simulink model "ModuleCooling"  (R2024b)
settings: Solver=VariableStepAuto  StartTime=0.0  StopTime=800  RelTol=1e-3
PostLoadFcn:
  | pouchPackExample_param;
  | load Artemis150mphCurrent_TS.mat;
undefined symbols (not defined in the file or in its folder): battery_builder_rtmsupport, gcbh
libraries: fl_lib x7, nesl_utility x6, batt_lib x2, pouchPackExample_lib x1, SimscapeFluids_lib x1
settings Model: Creator=xiangchz  LastModifiedBy=xiangchz
settings OptimizationCC: ReuseModelBlockBuffer=off
settings RTWCC: GPUComputeCapability=3.5
settings SimscapeCC: SimscapeLogType=all

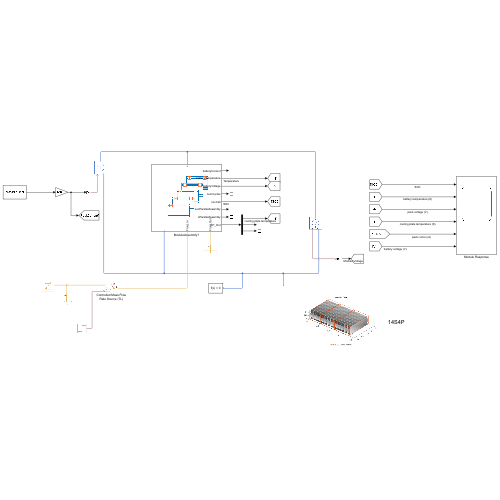
[thumbnail: Simulink's stored preview of the top-level diagram]
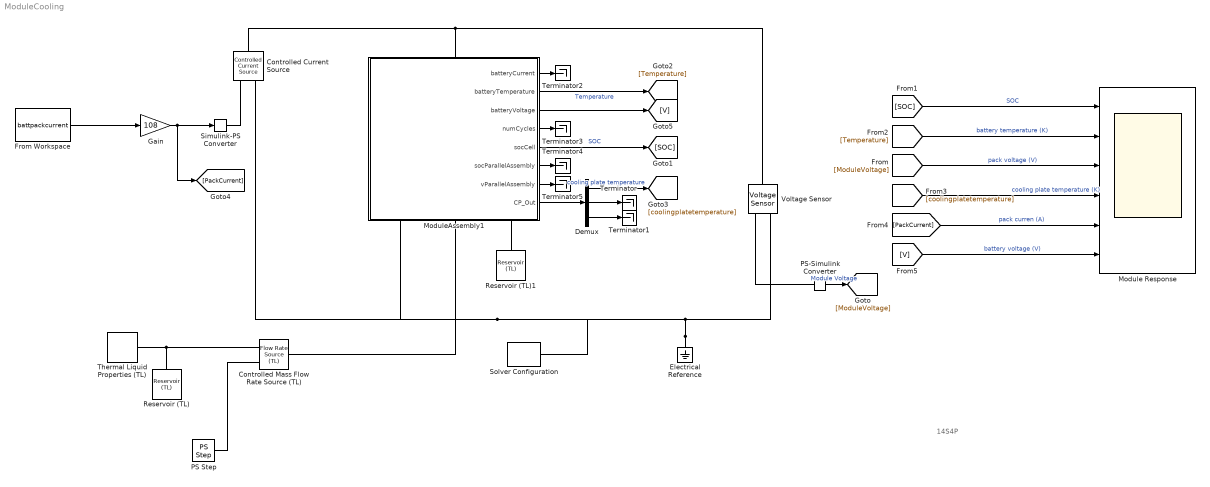
== system ModuleCooling ==
  note: 14S4P
  Controlled Current Source : fl_lib/Electrical/Electrical Sources/Controlled Current Source
  Controlled Mass Flow Rate Source (TL) : fl_lib/Thermal Liquid/Sources/Flow Rate Source (TL)  source_type=foundation.enum.constant_controlled.controlled  flow_type=foundation.enum.mass_volumetric_flow.mass  mass_flow=0 kg/s  volumetric_flow=0 m^3/s  power_spec=foundation.enum.power_spec.isentropic  area=0.01 m^2
  Demux : Demux  Outputs=[10 1 1]
  Electrical Reference : fl_lib/Electrical/Electrical Elements/Electrical Reference
  From Workspace : FromWorkspace  VariableName=battpackcurrent  OutputAfterFinalValue=Setting to zero
  Gain : Gain  Gain=108
  Module Response : Scope  NumInputPorts=6
  ModuleAssembly1 : Subsystem  LoadFcn=battery_builder_rtmsupport('loadfcn',gcbh);
      settings: CopyFcn=battery_builder_rtmsupport('copyfcn',gcbh);  PreCopyFcn=battery_builder_rtmsupport('precopyfcn',gcbh);  PreDeleteFcn=battery_builder_rtmsupport('predeletefcn',gcbh);  PortSchema="{\"entries\":[{\"content\":{\"sides\":[{\"content\":{\"connectorIds\":[\"LConn1\"]},\"type\":\"ConnectorPlacement.EquallySpacedRectSide\",\"uuid\":\"a5a584e8-f613-435c-beac-db0de62ed6e0\"},{\"content\":{\"connectorIds\":[\"RConn1\",\"RConn2\",\"RConn3\"],\"side\":\"RIGHT\"},\"type\":\"ConnectorPlacement.EquallySpacedRectSide\",\"uuid\":\"d51acd9b-f0fc-42a2-9d6d-d5cd10e7587e\"},{\"content\":{\"side\":\"TOP\"},\"type\":\"ConnectorPlacement.EquallySpacedRectSide\",\"uuid\":\"737671ea-5ed7-4c33-80c9-a3aa253c798a\"},{\"content\":{\"connectorIds\":[\"Out1\",\"Out2\",\"Out3\",\"Out4\",\"Out5\",\"Out6\",\"Out7\",\"Out8\"],\"side\":\"BOTTOM\"},\"type\":\"ConnectorPlacement.EquallySpacedRectSide\",\"uuid\":\"87a5caa8-fa5f-4d9a-a175-65997483afd1\"}]},\"type\":\"ConnectorPlacement.EquallySpacedConnector\",\"uuid\":\"0c8ecf39-6b75-42df-9e5b-e3923eef789f\"}],\"packageUris\":[\"http://schema.mathworks.com/mf0/Connector/R2020b\"],\"version\":\"1.0\"}"
      mask Display: image('$imagefile')
  PS Step : fl_lib/Physical Signals/Sources/PS Step  step_time=300 s  initial_value=0  final_value=0.03 kg/s
  PS-Simulink Converter : nesl_utility/PS-Simulink Converter  PhysicalDomain=network_engine_domain  SubClassName=ps_output  LeftPortType=input  RightPortType=output  PseudoPeriodic=off  Frequencies=[]  VectorFormat=inherit  Unit=inherit  AffineConversion=off
  Reservoir (TL) : fl_lib/Thermal Liquid/Elements/Reservoir (TL)  pressure_spec=foundation.enum.pressure_spec.atmospheric  reservoir_pressure=0.101325 MPa  reservoir_temperature=293.15 K  area=0.01 m^2
  Reservoir (TL)1 : fl_lib/Thermal Liquid/Elements/Reservoir (TL)  pressure_spec=foundation.enum.pressure_spec.atmospheric  reservoir_pressure=0.101325 MPa  reservoir_temperature=290 K  area=0.01 m^2
  Simulink-PS Converter : nesl_utility/Simulink-PS Converter  PhysicalDomain=network_engine_domain  SubClassName=ps_input  LeftPortType=input  RightPortType=output  PseudoPeriodic=off  Frequencies=[]  NoiseDistribution=none  NoiseParameters=[]  Unit=A  AffineConversion=off  FilteringAndDerivatives=provide  SimscapeFilterOrder=1  InputFilterTimeConstant=0.001  UdotUserProvided=0
  Solver Configuration : nesl_utility/Solver Configuration  PhysicalDomain=network_engine_domain  SubClassName=solver  LeftPortType=input  RightPortType=generic  Tones=[]  Harmonics=[]  SimulateNoise=off  Profile=off  UseLocalSampling=off  EnableSwitchedLinearOptims=on  FrequencyDomain=off  UseCCode=off  RelTol=0.001  AbsTol=0.001  MinStep=1e-09  ToWorkspace=off  RevertToSquareIcSolve=off  NumHomotopyIterations=100  PhasorMode=off  PhasorModeNumHarmonics=1  ConsistencySolver=NEWTON_XTOL_AFTER_FTOL  IndexReductionMethod=DerivativeReplacement  DoDC=off  ResidualTolerance=1e-09  ConsistencyTolSource=GLOBAL  ConsistencyAbsTol=0.001  ConsistencyRelTol=0.001  ConsistencyTolFactor=0.001  UseLocalSolver=off  LocalSolverChoice=NE_BACKWARD_EULER_ADVANCER  ResolveIndetEquations=on  FunctionEvalNumThread=1  LocalSolverSampleTime=0.001  DoFixedCost=off  MaxNonlinIter=3  MaxModeIter=2  ComputeImpulses=off  ImpulseIterations=2  LinearAlgebra=auto  LinearAlgebraNumThread=0  EquationFormulation=NE_TIME_EF  DelaysMemoryBudget=1024  AutomaticFiltering=on  FilteringTimeConstant=0.001  PartitionStorageMethod=AS_NEEDED  PartitionMemoryBudget=1024  PartitionMethod=ROBUST  MultibodyUseLocalSolver=off  MultibodyLocalSolverChoice=ODE1  MultibodyLocalSolverSampleTime=0.001
  Terminator{,1..5} (6 alike) : Terminator
  Thermal Liquid Properties (TL) : SimscapeFluids_lib/Thermal Liquid/Utilities/Thermal Liquid Properties (TL)  fluid_list=fluids.thermal_liquid.utilities.enum.thermal_liquid_fluid_list.water  concentration_param_EG=fluids.thermal_liquid.utilities.enum.thermal_liquid_concentration.volume_fraction  concentration_param_PG=fluids.thermal_liquid.utilities.enum.thermal_liquid_concentration.volume_fraction  c_mass_SW=3.5e-3  c_mass_EG=0.1  c_mass_PG=0.1  c_mass_GL=0.1  c_vol_EG=0.1  c_vol_PG=0.1  beta_const_EG=2.1791 GPa  beta_const_PG=2.1791 GPa  beta_const_GL=2.1791 GPa  p_min_EG=0.01 MPa  p_min_PG=0.01 MPa  p_min_GL=0.01 MPa  p_max_EG=50 MPa  p_max_PG=50 MPa  p_max_GL=50 MPa  p_atm=0.101325 MPa  properties_range_check=simscape.enum.assert.action.error
  Voltage Sensor : fl_lib/Electrical/Electrical Sensors/Voltage Sensor
  wires:
  ModuleAssembly1/8(CP_Out) -> Demux/1
  Demux/2 -> Terminator/1
  Demux/3 -> Terminator1/1
  PS-Simulink Converter/1 -> [ModuleVoltage]  "Module Voltage"
  [ModuleVoltage] -> Module Response/3  "pack voltage (V)"
  ModuleAssembly1/5(socCell) -> [SOC]  "SOC"
  [SOC] -> Module Response/1  "SOC"
  ModuleAssembly1/2(batteryTemperature) -> [Temperature]  "Temperature"
  [Temperature] -> Module Response/2  "battery temperature (K)"
  Demux/1 -> [coolingplatetemperature]  "cooling plate temperature"
  [coolingplatetemperature] -> Module Response/4  "cooling plate temperature (K)"
  Gain/1 -> Simulink-PS Converter/1, [PackCurrent]
  [PackCurrent] -> Module Response/5  "pack curren (A)"
  ModuleAssembly1/3(batteryVoltage) -> [V]
  [V] -> Module Response/6  "battery voltage (V)"
  From Workspace/1 -> Gain/1
  ModuleAssembly1/1(batteryCurrent) -> Terminator2/1
  ModuleAssembly1/4(numCycles) -> Terminator3/1
  ModuleAssembly1/6(socParallelAssembly) -> Terminator4/1
  ModuleAssembly1/7(vParallelAssembly) -> Terminator5/1
  connections:
  Voltage Sensor/LConn1 -- ModuleAssembly1/LConn1 -- Controlled Current Source/LConn1
  Electrical Reference/LConn1 -- ModuleAssembly1/RConn1 -- Controlled Current Source/RConn2 -- Solver Configuration/RConn1 -- Voltage Sensor/RConn2
  Voltage Sensor/RConn1 -- PS-Simulink Converter/LConn1
  ModuleAssembly1/RConn2 -- Controlled Mass Flow Rate Source (TL)/RConn1
  Reservoir (TL)/LConn1 -- Controlled Mass Flow Rate Source (TL)/LConn1 -- Thermal Liquid Properties (TL)/RConn1
  PS Step/RConn1 -- Controlled Mass Flow Rate Source (TL)/LConn2
  ModuleAssembly1/RConn3 -- Reservoir (TL)1/LConn1
  Simulink-PS Converter/RConn1 -- Controlled Current Source/RConn1

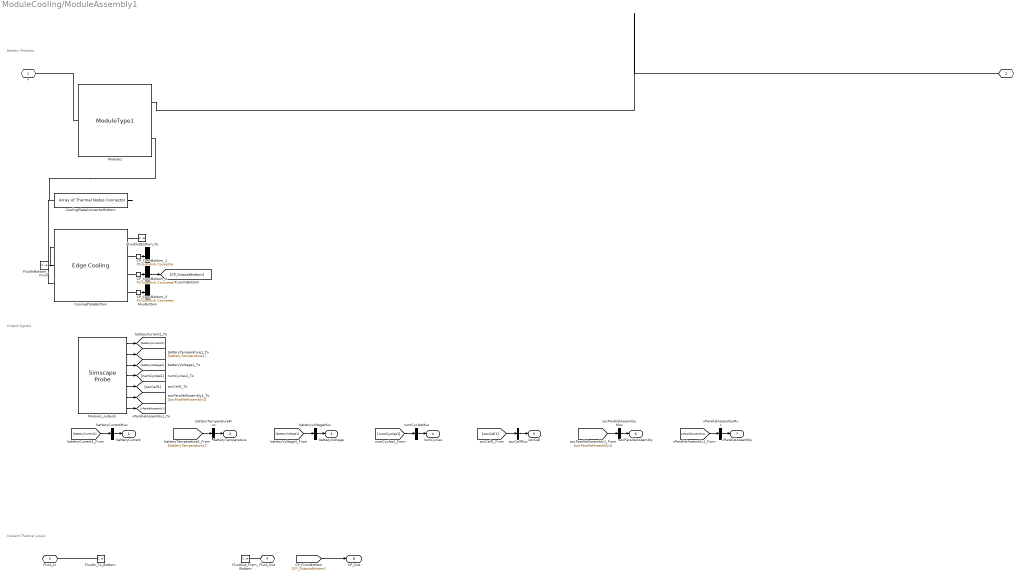
== system ModuleCooling/ModuleAssembly1 ==
  note: Coolant Thermal Liquid
  note: Output Signals
  note: Battery Modules
  CP_ConvBottom_1 : nesl_utility/PS-Simulink Converter  PhysicalDomain=network_engine_domain  SubClassName=ps_output  LeftPortType=input  RightPortType=output  PseudoPeriodic=off  Frequencies=[]  VectorFormat=inherit  Unit=inherit  AffineConversion=off
  CP_ConvBottom_2 : nesl_utility/PS-Simulink Converter  PhysicalDomain=network_engine_domain  SubClassName=ps_output  LeftPortType=input  RightPortType=output  PseudoPeriodic=off  Frequencies=[]  VectorFormat=inherit  Unit=inherit  AffineConversion=off
  CP_ConvBottom_3 : nesl_utility/PS-Simulink Converter  PhysicalDomain=network_engine_domain  SubClassName=ps_output  LeftPortType=input  RightPortType=output  PseudoPeriodic=off  Frequencies=[]  VectorFormat=inherit  Unit=inherit  AffineConversion=off
  CoolingPlateBottom : batt_lib/Thermal/Edge Cooling  plateConnectivity=simscape.battery.enum.thermal.coolingPlateConnectivity.singleSided  numBattThermalNodes1=CoolingPlateBottom.numBattThermalNodes1  dimensionThermalNodes1=CoolingPlateBottom.dimensionThermalNodes1  locationThermalNodes1=CoolingPlateBottom.locationThermalNodes1  numBattThermalNodes2=1  dimensionThermalNodes2=ones(1, 2)  locationThermalNodes2=ones(1, 2)  plateDimX=CoolingPlateBottom.plateDimX  plateDimY=CoolingPlateBottom.plateDimY  plateTh=CoolingPlateBottom.plateTh m  plateThCond=CoolingPlateBottom.plateThCond W/(K*m)  plateDen=CoolingPlateBottom.plateDen kg/m^3  plateCp=CoolingPlateBottom.plateCp J/(K*kg)  plateTemp_ini=CoolingPlateBottom.plateTemp_ini K  Re_lam=CoolingPlateBottom.Re_lam  Re_tur=CoolingPlateBottom.Re_tur  Nu_lam=CoolingPlateBottom.Nu_lam  length_add=CoolingPlateBottom.length_add m  shape_factor=CoolingPlateBottom.shape_factor  selectEdgeOrientation=simscape.battery.enum.thermal.coolingEdgeDirection.alongX0  channelDia=CoolingPlateBottom.channelDia m  channelArea=CoolingPlateBottom.channelArea m^2  roughnessPipe=CoolingPlateBottom.roughnessPipe m
      settings: InternalSimscapePortConfiguration="{\"Bottom\":[],\"Left\":[{\"id\":\"fluid_in\",\"label\":\"fluid_in\",\"type\":\"foundation.thermal_liquid.thermal_liquid\"}],\"Right\":[{\"id\":\"fluid_out\",\"label\":\"fluid_out\",\"type\":\"foundation.thermal_liquid.thermal_liquid\"},{\"id\":\"plotPlateT\",\"label\":\"Tp\",\"type\":\"output\"},{\"id\":\"tempSensor\",\"label\":\"dT\",\"type\":\"output\"},{\"id\":\"presSensor\",\"label\":\"dP\",\"type\":\"output\"}],\"Top\":[{\"id\":\"Side1\",\"label\":\"Surf1\",\"type\":\"foundation.thermal.thermal\"}]}"
  CoolingPlateConnectorBottom : batt_lib/Thermal/Array of Thermal Nodes Connector  numInputConnections=1  concatenateDimension=2  complementaryDimensionsSize=1  inNode1NumElements=3  inNode2NumElements=1  inNode3NumElements=1  inNode4NumElements=1  inNode5NumElements=1  inNode6NumElements=1  inNode7NumElements=1  inNode8NumElements=1  inNode9NumElements=1  inNode10NumElements=1  inNode11NumElements=1  inNode12NumElements=1  inNode13NumElements=1  inNode14NumElements=1  inNode15NumElements=1  inNode16NumElements=1  inNode17NumElements=1  inNode18NumElements=1  inNode19NumElements=1  inNode20NumElements=1  inNode21NumElements=1  inNode22NumElements=1  inNode23NumElements=1  inNode24NumElements=1  inNode25NumElements=1  inNode26NumElements=1  inNode27NumElements=1  inNode28NumElements=1  inNode29NumElements=1  inNode30NumElements=1  inNode31NumElements=1  inNode32NumElements=1  inNode33NumElements=1  inNode34NumElements=1  inNode35NumElements=1  inNode36NumElements=1  inNode37NumElements=1  inNode38NumElements=1  inNode39NumElements=1  inNode40NumElements=1  inNode41NumElements=1  inNode42NumElements=1  inNode43NumElements=1  inNode44NumElements=1  inNode45NumElements=1  inNode46NumElements=1  inNode47NumElements=1  inNode48NumElements=1  inNode49NumElements=1  inNode50NumElements=1
      settings: InternalSimscapePortConfiguration="{\"Bottom\":[{\"id\":\"outConn\",\"label\":\"outConn\",\"type\":\"foundation.thermal.thermal\"}],\"Left\":[],\"Right\":[],\"Top\":[{\"id\":\"inConn1\",\"label\":\"inConn1\",\"type\":\"foundation.thermal.thermal\"}]}"
  FluidInBottom_From : ConnectionLabel  Label=FluidIn_To_Bottom
  FluidIn_To_Bottom : ConnectionLabel  Label=FluidIn_To_Bottom
  FluidOutBottom_To : ConnectionLabel  Label=FluidOut_From_Bottom
  FluidOut_From_Bottom : ConnectionLabel  Label=FluidOut_From_Bottom
  Module1 : pouchPackExample_lib/Modules/ModuleType1  BatteryCapacityCell=ModuleType1.BatteryCapacityCell A*hr  ExtrapolationMethodCell=simscape.enum.extrapolation.nearest  SOCBreakpointsCell=ModuleType1.SOCBreakpointsCell  TemperatureBreakpointsCell=ModuleType1.TemperatureBreakpointsCell K  OpenCircuitVoltageThermalCell=ModuleType1.OpenCircuitVoltageThermalCell V  VoltageRangeCell=ModuleType1.VoltageRangeCell V  ResistanceSOCBreakpointsCell=ModuleType1.ResistanceSOCBreakpointsCell  ResistanceTemperatureBreakpointsCell=ModuleType1.ResistanceTemperatureBreakpointsCell K  R0ThermalCell=ModuleType1.R0ThermalCell Ohm  R1ThermalCell=ModuleType1.R1ThermalCell Ohm  Tau1ThermalCell=ModuleType1.Tau1ThermalCell s  BatteryThermalMassCell=ModuleType1.BatteryThermalMassCell J/K  CoolantResistance=ModuleType1.CoolantResistance K/W  P=4  S=14  SeriesGrouping=[4, 5, 5]  ParallelGrouping=[1, 1, 1]  socCell_specify=on  socCell_priority=High  socCell=Module1.socCell  socCell_nominal_specify=off  socCell_nominal_value=1  socCell_nominal_unit=1  numCycles_specify=on  numCycles_priority=High  numCycles=Module1.numCycles  numCycles_nominal_specify=off  numCycles_nominal_value=1  numCycles_nominal_unit=1  batteryVoltage_specify=on  batteryVoltage_priority=None  batteryVoltage=Module1.batteryVoltage V  batteryVoltage_nominal_specify=off  batteryVoltage_nominal_value=1  batteryVoltage_nominal_unit=V  batteryCurrent_specify=on  batteryCurrent_priority=None  batteryCurrent=Module1.batteryCurrent A  batteryCurrent_nominal_specify=off  batteryCurrent_nominal_value=1  batteryCurrent_nominal_unit=A  batteryTemperature_specify=on  batteryTemperature_priority=High  batteryTemperature=Module1.batteryTemperature K  batteryTemperature_nominal_specify=off  batteryTemperature_nominal_value=1  batteryTemperature_nominal_unit=K  vParallelAssembly_specify=on  vParallelAssembly_priority=None  vParallelAssembly=Module1.vParallelAssembly V  vParallelAssembly_nominal_specify=off  vParallelAssembly_nominal_value=1  vParallelAssembly_nominal_unit=V  socParallelAssembly_specify=on  socParallelAssembly_priority=None  socParallelAssembly=Module1.socParallelAssembly  socParallelAssembly_nominal_specify=off  socParallelAssembly_nominal_value=1  socParallelAssembly_nominal_unit=1
      settings: InternalSimscapePortConfiguration="{\"Bottom\":[{\"id\":\"n\",\"label\":\"-\",\"type\":\"foundation.electrical.electrical\"},{\"id\":\"BottomExtClnt\",\"label\":\"CPB\",\"type\":\"foundation.thermal.thermal\"}],\"Left\":[],\"Right\":[],\"Top\":[{\"id\":\"p\",\"label\":\"+\",\"type\":\"foundation.electrical.electrical\"}]}"
  Module1_outputs : SimscapeProbe  BoundBlock=471  Variables={batteryCurrent, batteryTemperature, batteryVoltage, numCycles, socCell, socParallelAssembly, vParallelAssembly}
  MuxBottom : Mux  Inputs=3
  batteryCurrentMux : Mux  Inputs=1
  batteryTemperatureMux : Mux  Inputs=1
  batteryVoltageMux : Mux  Inputs=1
  numCyclesMux : Mux  Inputs=1
  socCellMux : Mux  Inputs=1
  socParallelAssemblyMux : Mux  Inputs=1
  vParallelAssemblyMux : Mux  Inputs=1
  + : PMIOPort  Side=Left
  - : PMIOPort  Port=2  Side=Right
  Fluid_In : PMIOPort  Port=3  Side=Right  ConnectionType=Connection: foundation.thermal_liquid.thermal_liquid
  Fluid_Out : PMIOPort  Port=4  Side=Right  ConnectionType=Connection: foundation.thermal_liquid.thermal_liquid
  batteryCurrent : Outport
  batteryTemperature : Outport  Port=2
  batteryVoltage : Outport  Port=3
  numCycles : Outport  Port=4
  socCell : Outport  Port=5
  socParallelAssembly : Outport  Port=6
  vParallelAssembly : Outport  Port=7
  CP_Out : Outport  Port=8
  wires:
  [CP_OutputsBottom] -> CP_Out/1
  MuxBottom/1 -> [CP_OutputsBottom]
  CP_ConvBottom_3/1 -> MuxBottom/3
  CP_ConvBottom_2/1 -> MuxBottom/2
  CP_ConvBottom_1/1 -> MuxBottom/1
  [vParallelAssembly1] -> vParallelAssemblyMux/1
  vParallelAssemblyMux/1 -> vParallelAssembly/1
  Module1_outputs/7 -> [vParallelAssembly1]
  [socParallelAssembly1] -> socParallelAssemblyMux/1
  socParallelAssemblyMux/1 -> socParallelAssembly/1
  Module1_outputs/6 -> [socParallelAssembly1]
  [socCell1] -> socCellMux/1
  socCellMux/1 -> socCell/1
  Module1_outputs/5 -> [socCell1]
  [numCycles1] -> numCyclesMux/1
  numCyclesMux/1 -> numCycles/1
  Module1_outputs/4 -> [numCycles1]
  [batteryVoltage1] -> batteryVoltageMux/1
  batteryVoltageMux/1 -> batteryVoltage/1
  Module1_outputs/3 -> [batteryVoltage1]
  [batteryTemperature1] -> batteryTemperatureMux/1
  batteryTemperatureMux/1 -> batteryTemperature/1
  Module1_outputs/2 -> [batteryTemperature1]
  [batteryCurrent1] -> batteryCurrentMux/1
  batteryCurrentMux/1 -> batteryCurrent/1
  Module1_outputs/1 -> [batteryCurrent1]
  connections:
  CoolingPlateBottom/RConn4 -- CP_ConvBottom_3/LConn1
  CoolingPlateBottom/RConn3 -- CP_ConvBottom_2/LConn1
  CoolingPlateBottom/RConn2 -- CP_ConvBottom_1/LConn1
  CoolingPlateBottom/RConn1 -- FluidOutBottom_To/LConn1
  FluidInBottom_From/LConn1 -- CoolingPlateBottom/LConn1
  Fluid_Out/RConn1 -- FluidOut_From_Bottom/LConn1
  FluidIn_To_Bottom/LConn1 -- Fluid_In/RConn1
  CoolingPlateConnectorBottom/RConn1 -- CoolingPlateBottom/LConn2
  CoolingPlateConnectorBottom/LConn1 -- Module1/RConn2
  Module1/RConn1 -- -/RConn1
  Module1/LConn1 -- +/RConn1
